simulink model "APV_ensemble_training"  (R2022a)
settings: Solver=VariableStepAuto  StartTime=0.0  StopTime=Tf  RelTol=1e-3  AbsTol=1e-4
InitFcn:
  | % show(map);
  | if doTraining == 0
  | setOccupied(map, 1:46);
  | setFree(map, freeSpotIndex);
  | end
values from neighbouring files (symbols this model uses):
  centerToRear = 1.343    [ParkingLotEnvironment.m]    (also in autoParkingValetParams3D.m)
  lidarTol = 0.2    [autoParkingValetParams3D.m]
  map = evalin('base',obj.MapObject)    [Camera.m]    (also in LIDARSensor.m = evalin('base', this.MapObject); ParkingLot2DVisualizer.m)
  maxLidarDist = 6    [autoParkingValetParams3D.m]
  numSensors = numel(lidar)    [ParkingLotEnvironment.m]    (also in autoParkingValetParams3D.m = 12)
  pTracking = 10    [createMPCForParking3D.m]
  speedMax = 2    [autoParkingValetParams3D.m]
  steerMax = pi/4    (= 0.785398163397)    [autoParkingValetParams3D.m]
  terrTol = deg2rad(10)    [autoParkingValetParams3D.m]
  trainXBounds = map.TrainingZoneXLimits    [autoParkingValetParams3D.m]
  trainYBounds = map.TrainingZoneYLimits    [autoParkingValetParams3D.m]
  Ts = 0.1    [createMPCForParking3D.m]
  xBounds = map.XLimits    [autoParkingValetParams3D.m]
  Xref = createReferenceTrajectory(Ts,Tf,freeSpotIndex)    [createMPCForParking3D.m]    (also in createReferenceTrajectory.m = [xRef(1:p,:);repmat(xRef(end,:),Tsteps-p,1)])
  xyerrTol = 0.75    [autoParkingValetParams3D.m]
  yBounds = map.YLimits    [autoParkingValetParams3D.m]
undefined symbols (not defined in the file or in its folder): actionTable, actionUB, collisionGain, distWeight, doTraining, egoInitialPose, egoTargetPose, freeSpotIndex, isTerminate, lidarGain, orientWeight, parkGain, rewardToIndex, rewardUB1, rewardUB2, stableWeight, stateTable, Tf, tranTable
libraries: rllib x10, mpclib x2, simulink x1, robotmobilelib x1, simulink_extras x1, sim3dlib x1, sim3dautolib x1
settings Model: PacingRate=0.089000  Creator=The MathWorks, Inc.  LastModifiedBy=momentumlab
settings SolverCC: AutoScaleAbsTol=off  AlgebraicLoopSolver=TrustRegion  MinimalZcImpactIntegration=on  MaxZcPerStep=1
settings DataIOCC: ReturnWorkspaceOutputs=off
settings DebuggingCC: UnconnectedInputMsg=warning  UnconnectedOutputMsg=warning  UnconnectedLineMsg=warning  SFMachineParentedDataDiag=warning
settings RTWCC: DLArmComputeVersion=19.05

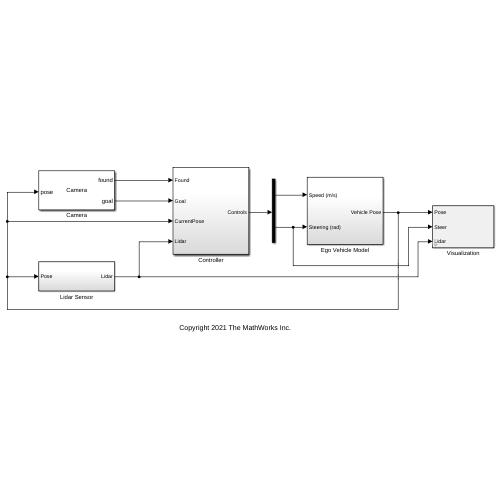
[thumbnail: Simulink's stored preview of the top-level diagram]
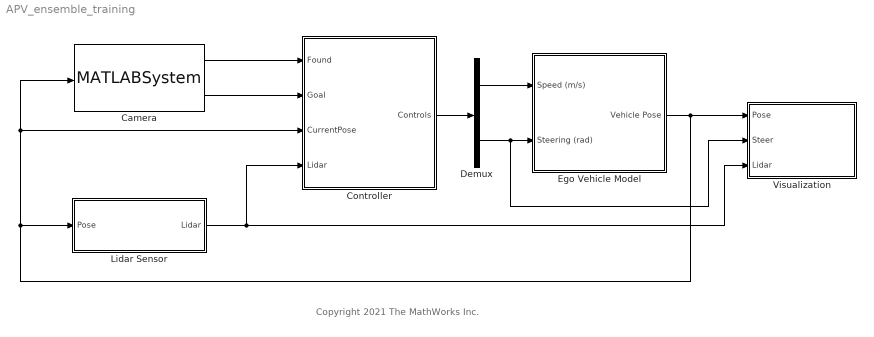
== system APV_ensemble_training ==
  note: Copyright 2021 The MathWorks Inc.
  Camera : MATLABSystem  System=Camera  MaxDepth=cameraDepth  MaxViewAngle=cameraViewAngle  MapObject=map
      mask Type: Camera
      mask Display:
      | disp('Camera');
      | port_label('input',1,'pose');
      | port_label('output',1,'found');
      | port_label('output',2,'goal');
  Controller : Subsystem
  Demux : Demux  Outputs=2
  Ego Vehicle Model : Subsystem
  Lidar Sensor : Subsystem
  Visualization : Subsystem  mask{doViz=Off, doVizUnreal=Off}
      mask prompts: doViz "2D Visualization"; doVizUnreal "Unreal Engine Visualization"
      mask TypeOptions doViz: Parking Lot 2D Visualization/doViz
      mask TypeOptions doVizUnreal: Unreal Engine Visualization/doVizUnreal
      mask DialogControl DescTextVar Prompt: Specify visualization options.
  wires:
  Demux/1 -> Ego Vehicle Model/1(Speed (m/s))
  Demux/2 -> Visualization/2(Steer), Ego Vehicle Model/2(Steering (rad))
  Lidar Sensor/1(Lidar) -> Visualization/3(Lidar), Controller/4(Lidar)
  Camera/1 -> Controller/1(Found)
  Camera/2 -> Controller/2(Goal)
  Controller/1(Controls) -> Demux/1
  Ego Vehicle Model/1(Vehicle Pose) -> Camera/1, Controller/3(CurrentPose), Lidar Sensor/1(Pose), Visualization/1(Pose)

== system APV_ensemble_training/Controller ==
  Found : Inport
  Goal : Inport  Port=2
  CurrentPose : Inport  Port=3
  Lidar : Inport  Port=4
  MPC Tracking Controller : Subsystem
  Merge : Merge
  RL Controller : Subsystem
  Vehicle Mode : Subsystem
  Controls : Outport
  wires:
  Merge/1 -> Controls/1
  CurrentPose/1 -> RL Controller/2(CurrentPose), MPC Tracking Controller/1(States)
  Vehicle Mode/3(TargetPose) -> RL Controller/1(Target)
  Lidar/1 -> RL Controller/3(Lidar)
  RL Controller/1(Actions) -> Merge/2
  MPC Tracking Controller/1(Controls) -> Merge/1
  Goal/1 -> Vehicle Mode/2(Goal)
  Found/1 -> Vehicle Mode/1(Found)
  Vehicle Mode/1(Search) -> MPC Tracking Controller/Enable
  Vehicle Mode/2(Park) -> RL Controller/Enable

== system APV_ensemble_training/Ego Vehicle Model ==
  Speed (m/s) : Inport
  Steering (rad) : Inport  Port=2
  Bicycle Kinematic Model : robotmobilelib/Bicycle Kinematic Model  VehicleInputs=Vehicle Speed & Steering Angle  WheelBase=map.centerToRear+map.centerToFront  VehicleSpeedRange=[-5, 5]  MaxSteeringAngle=steerMax  InitialState=egoInitialPose  SimulateUsing=Interpreted execution
      settings: SourceProductBaseCode=RO
  Demux : Demux  Outputs=3
  Ego Vehicle Pose : Scope  NumInputPorts=3
  Terminator : Terminator
  Vehicle Pose : Outport
  wires:
  Demux/3 -> Ego Vehicle Pose/3  "theta (rad)"
  Bicycle Kinematic Model/1 -> Demux/1, Vehicle Pose/1
  Demux/1 -> Ego Vehicle Pose/1  "x (m)"
  Bicycle Kinematic Model/2 -> Terminator/1
  Demux/2 -> Ego Vehicle Pose/2  "y (m)"
  Speed (m/s)/1 -> Bicycle Kinematic Model/1
  Steering (rad)/1 -> Bicycle Kinematic Model/2

== system APV_ensemble_training/Lidar Sensor ==
  Pose : Inport
  Demux : Demux  Outputs=3
  MATLAB System : MATLABSystem  System=LIDARSensor  MapObject=map  CarGeometry=map.VehicleDimensions  MaxDistance=maxLidarDist  SensorResolution=numSensors  ShowLIDARPlot=0  PlotLimits=[ xBounds yBounds ]
      mask Type: LIDARSensor
      mask Display:
      | disp('LIDARSensor');
      | port_label('input',1,'botx');
      | port_label('input',2,'boty');
      | port_label('input',3,'theta');
      | port_label('output',1,'d');
  Subsystem : Subsystem
  Lidar : Outport
  wires:
  Pose/1 -> Demux/1
  MATLAB System/1 -> Lidar/1
  Subsystem/1(centerX) -> MATLAB System/1
  Demux/2 -> Subsystem/2(currY)
  Demux/3 -> MATLAB System/3, Subsystem/3(theta)
  Demux/1 -> Subsystem/1(currX)
  Subsystem/2(centerY) -> MATLAB System/2

== system APV_ensemble_training/Visualization ==
  Pose : Inport
  Steer : Inport  Port=2
  Lidar : Inport  Port=3
  Parking Lot 2D Visualization : Subsystem  Variant=on  VariantControlMode=label  VariantControl=Choice  LabelModeActiveChoice=VizOff  mask{doViz=Off}
      mask prompts: doViz "2D Visualization"
      mask init:
      | choice = get_param(gcb,'doViz');
      | vssBlk = gcb;
      | if strcmp(choice,'On')
      |     set_param(vssBlk, 'LabelModeActiveChoice', 'VizOn');
      | else
      |     set_param(vssBlk, 'LabelModeActiveChoice', 'VizOff');
      | end
      mask TypeOptions doViz: On | Off
      mask DialogControl DescTextVar Tooltip: {"textId":"","text":""}
  Unreal Engine Visualization : Subsystem  Variant=on  VariantControlMode=label  VariantControl=Choice  LabelModeActiveChoice=UnrealOff  mask{doVizUnreal=Off}
      mask prompts: doVizUnreal "Unreal Engine Visualization"
      mask init:
      | choice = get_param(gcb,'doVizUnreal');
      | vssBlk = gcb;
      | if strcmp(choice,'On')
      |     set_param(vssBlk, 'LabelModeActiveChoice', 'UnrealOn');
      | else
      |     set_param(vssBlk, 'LabelModeActiveChoice', 'UnrealOff');
      | end
      mask TypeOptions doVizUnreal: On | Off
      mask DialogControl DescTextVar Tooltip: {"textId":"","text":""}
  wires:
  Pose/1 -> Unreal Engine Visualization/1(Pose), Parking Lot 2D Visualization/1(Pose)
  Steer/1 -> Parking Lot 2D Visualization/2(Steer)
  Lidar/1 -> Parking Lot 2D Visualization/3(Lidar)

== system APV_ensemble_training/Controller/MPC Tracking Controller ==
  States : Inport
  Enable : EnablePort  StatesWhenEnabling=reset
  Variant Subsystem : Subsystem  Variant=on  VariantControlMode=label  LabelModeActiveChoice=Choice_1  mask{choice=Adaptive MPC}
      mask init:
      | choice = get_param(gcb,'choice');
      | vssBlk = gcb;
      | oldVariant = get_param(gcb,'LabelModeActiveChoice');
      | if strcmp(choice,'Adaptive MPC')
      |     
      |     set_param(vssBlk, 'LabelModeActiveChoice', 'Choice_1');
      | else
      |     
      |     set_param(vssBlk, 'LabelModeActiveChoice', 'Choice_2');
      | end
      mask TypeOptions choice: Adaptive MPC | Nonlinear MPC
  Controls : Outport
  wires:
  States/1 -> Variant Subsystem/1(states)
  Variant Subsystem/1(controls) -> Controls/1

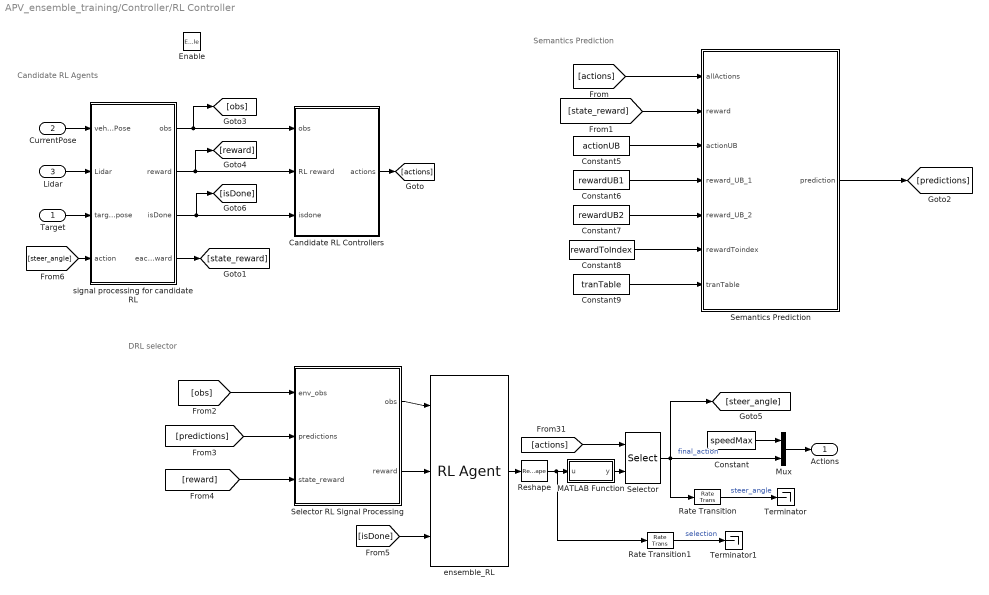
== system APV_ensemble_training/Controller/RL Controller ==
  note: Semantics Prediction
  note: Candidate RL Agents
  note: DRL selector
  Target : Inport
  CurrentPose : Inport  Port=2
  Lidar : Inport  Port=3
  Enable : EnablePort  StatesWhenEnabling=reset
  Candidate RL Controllers : Subsystem
  Constant : Constant  Value=speedMax
  Constant5 : Constant  Value=actionUB
  Constant6 : Constant  Value=rewardUB1
  Constant7 : Constant  Value=rewardUB2
  Constant8 : Constant  Value=rewardToIndex
  Constant9 : Constant  Value=tranTable
  MATLAB Function : MATLAB Function  TreatAsAtomicUnit=on
  Mux : Mux  Inputs=2
  Rate Transition : RateTransition  OutPortSampleTime=Ts_sample
  Rate Transition1 : RateTransition  OutPortSampleTime=Ts_sample
  Reshape : Reshape
  Selector : Selector  IndexOptions=Index vector (port)  Indices=[1 3]  OutputSizes=1
  Selector RL Signal Processing : Subsystem
  Semantics Prediction : Subsystem
  Terminator : Terminator
  Terminator1 : Terminator
  ensemble_RL : rllib/RL Agent  Agent=agentEnsemble  ExternalActionAsInput=off  ProvideLastAction=off  ProvideCumRwd=off  TreatAsDirectFeedthrough=on  UseStrictObservationDataTypes=off
  signal processing for candidate RL : Subsystem
  Actions : Outport
  wires:
  signal processing for candidate RL/1(obs) -> Candidate RL Controllers/1(obs), [obs]
  signal processing for candidate RL/2(reward) -> Candidate RL Controllers/2(RL reward), [reward]
  CurrentPose/1 -> signal processing for candidate RL/1(vehiclePose)
  Target/1 -> signal processing for candidate RL/3(targetpose)
  Lidar/1 -> signal processing for candidate RL/2(Lidar)
  Constant/1 -> Mux/1
  Mux/1 -> Actions/1
  signal processing for candidate RL/3(isDone) -> [isDone], Candidate RL Controllers/3(isdone)
  Rate Transition/1 -> Terminator/1  "steer_angle"
  Constant6/1 -> Semantics Prediction/4(reward_UB_1)
  Constant7/1 -> Semantics Prediction/5(reward_UB_2)
  Constant5/1 -> Semantics Prediction/3(actionUB)
  Constant9/1 -> Semantics Prediction/7(tranTable)
  [actions] -> Semantics Prediction/1(allActions)
  Constant8/1 -> Semantics Prediction/6(rewardToindex)
  Semantics Prediction/1(prediction) -> [predictions]
  [state_reward] -> Semantics Prediction/2(reward)
  Candidate RL Controllers/1(actions) -> [actions]
  [isDone] -> ensemble_RL/3
  Reshape/1 -> Rate Transition1/1, MATLAB Function/1(u)
  Selector/1 -> Rate Transition/1, Mux/2, [steer_angle]  "final_action"
  [predictions] -> Selector RL Signal Processing/2(predictions)
  Selector RL Signal Processing/2(reward) -> ensemble_RL/2
  [actions] -> Selector/1
  Selector RL Signal Processing/1(obs) -> ensemble_RL/1
  [obs] -> Selector RL Signal Processing/1(env_obs)
  [reward] -> Selector RL Signal Processing/3(state_reward)
  signal processing for candidate RL/4(each_reward) -> [state_reward]
  [steer_angle] -> signal processing for candidate RL/4(action)
  Rate Transition1/1 -> Terminator1/1  "selection"
  ensemble_RL/1 -> Reshape/1
  MATLAB Function/1(y) -> Selector/2

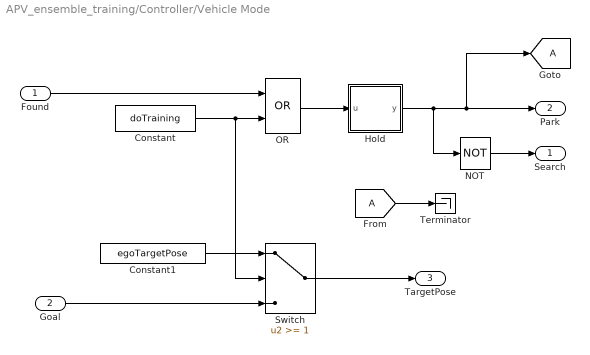
== system APV_ensemble_training/Controller/Vehicle Mode ==
  Found : Inport
  Goal : Inport  Port=2
  Constant : Constant  Value=doTraining
  Constant1 : Constant  Value=egoTargetPose
  From : From  TagVisibility=global
  Goto : Goto  TagVisibility=global
  Hold : Subsystem
  NOT : Logic  Operator=NOT  AllPortsSameDT=off  OutDataTypeStr=boolean
  OR : Logic  Operator=OR  AllPortsSameDT=off  OutDataTypeStr=boolean
  Switch : Switch  Threshold=1  SaturateOnIntegerOverflow=off  InputSameDT=off
  Terminator : Terminator
  Search : Outport
  Park : Outport  Port=2
  TargetPose : Outport  Port=3
  wires:
  Found/1 -> OR/1
  OR/1 -> Hold/1(u)
  NOT/1 -> Search/1
  Hold/1(y) -> Goto/1, Park/1, NOT/1
  Constant1/1 -> Switch/1
  Switch/1 -> TargetPose/1
  Constant/1 -> Switch/2, OR/2
  Goal/1 -> Switch/3
  From/1 -> Terminator/1

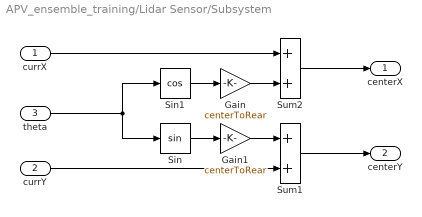
== system APV_ensemble_training/Lidar Sensor/Subsystem ==
  currX : Inport
  currY : Inport  Port=2
  theta : Inport  Port=3
  Gain : Gain  Gain=centerToRear
  Gain1 : Gain  Gain=centerToRear
  Sin : Trigonometry
  Sin1 : Trigonometry  Operator=cos
  Sum1 : Sum
  Sum2 : Sum
  centerX : Outport
  centerY : Outport  Port=2
  wires:
  Sum1/1 -> centerY/1
  currY/1 -> Sum1/2
  theta/1 -> Sin/1, Sin1/1
  Sin/1 -> Gain1/1
  Sin1/1 -> Gain/1
  currX/1 -> Sum2/1
  Sum2/1 -> centerX/1
  Gain/1 -> Sum2/2
  Gain1/1 -> Sum1/1

== system APV_ensemble_training/Visualization/Parking Lot 2D Visualization ==
  Pose : Inport
  Steer : Inport  Port=2
  Lidar : Inport  Port=3
  Off : Subsystem  VariantControl=VizOff
  On : Subsystem  VariantControl=VizOn

== system APV_ensemble_training/Visualization/Unreal Engine Visualization ==
  Pose : Inport
  Off : Subsystem  VariantControl=UnrealOff
  On : Subsystem  VariantControl=UnrealOn

== system APV_ensemble_training/Controller/MPC Tracking Controller/Variant Subsystem ==
  note: 1) Add Subsystem or Model blocks as valid variant choices.
      | 2) You cannot connect blocks at this level. At simulation, connectivity is automatically
      | determined, based on the active variant and port name matching.
  states : Inport
  Adaptive MPC : Subsystem  VariantControl=Choice_1
  Nonlinear MPC : Subsystem  VariantControl=Choice_2
  controls : Outport

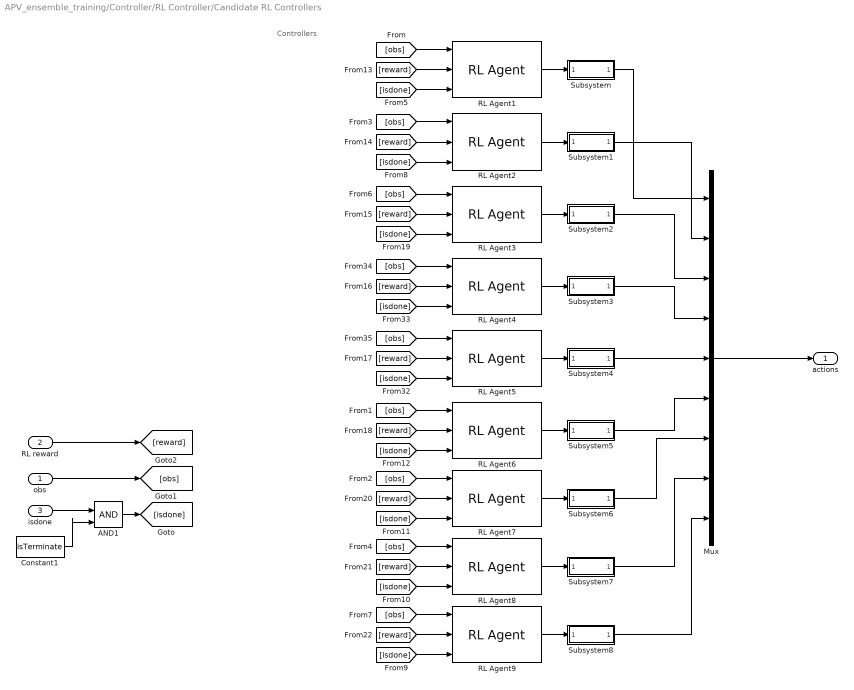
== system APV_ensemble_training/Controller/RL Controller/Candidate RL Controllers ==
  note: Controllers
  obs : Inport
  RL reward : Inport  Port=2
  isdone : Inport  Port=3
  AND1 : Logic  IconShape=distinctive  AllPortsSameDT=off  OutDataTypeStr=boolean
  Constant1 : Constant  Value=isTerminate
  Mux : Mux  Inputs=9
  RL Agent1 : rllib/RL Agent  Agent=agent1  ExternalActionAsInput=off  ProvideLastAction=off  ProvideCumRwd=off  TreatAsDirectFeedthrough=on  UseStrictObservationDataTypes=off
  RL Agent2 : rllib/RL Agent  Agent=agent2  ExternalActionAsInput=off  ProvideLastAction=off  ProvideCumRwd=off  TreatAsDirectFeedthrough=on  UseStrictObservationDataTypes=off
  RL Agent3 : rllib/RL Agent  Agent=agent3  ExternalActionAsInput=off  ProvideLastAction=off  ProvideCumRwd=off  TreatAsDirectFeedthrough=on  UseStrictObservationDataTypes=off
  RL Agent4 : rllib/RL Agent  Agent=agent3  ExternalActionAsInput=off  ProvideLastAction=off  ProvideCumRwd=off  TreatAsDirectFeedthrough=on  UseStrictObservationDataTypes=off
  RL Agent5 : rllib/RL Agent  Agent=agent3  ExternalActionAsInput=off  ProvideLastAction=off  ProvideCumRwd=off  TreatAsDirectFeedthrough=on  UseStrictObservationDataTypes=off
  RL Agent6 : rllib/RL Agent  Agent=agent6  ExternalActionAsInput=off  ProvideLastAction=off  ProvideCumRwd=off  TreatAsDirectFeedthrough=on  UseStrictObservationDataTypes=off
  RL Agent7 : rllib/RL Agent  Agent=agent7  ExternalActionAsInput=off  ProvideLastAction=off  ProvideCumRwd=off  TreatAsDirectFeedthrough=on  UseStrictObservationDataTypes=off
  RL Agent8 : rllib/RL Agent  Agent=agent8  ExternalActionAsInput=off  ProvideLastAction=off  ProvideCumRwd=off  TreatAsDirectFeedthrough=on  UseStrictObservationDataTypes=off
  RL Agent9 : rllib/RL Agent  Agent=agent9  ExternalActionAsInput=off  ProvideLastAction=off  ProvideCumRwd=off  TreatAsDirectFeedthrough=on  UseStrictObservationDataTypes=off
  Subsystem : Subsystem
  Subsystem1 : Subsystem
  Subsystem2 : Subsystem
  Subsystem3 : Subsystem
  Subsystem4 : Subsystem
  Subsystem5 : Subsystem
  Subsystem6 : Subsystem
  Subsystem7 : Subsystem
  Subsystem8 : Subsystem
  actions : Outport
  wires:
  [obs] -> RL Agent7/1
  [obs] -> RL Agent4/1
  [obs] -> RL Agent3/1
  Subsystem3/1(action) -> Mux/4
  [obs] -> RL Agent1/1
  [isdone] -> RL Agent1/3
  [obs] -> RL Agent2/1
  [obs] -> RL Agent5/1
  RL Agent1/1 -> Subsystem/1(rlOut)
  [isdone] -> RL Agent8/3
  [isdone] -> RL Agent6/3
  Subsystem/1(action) -> Mux/1
  RL Agent6/1 -> Subsystem5/1(rlOut)
  Subsystem4/1(action) -> Mux/5
  RL Agent3/1 -> Subsystem2/1(rlOut)
  [isdone] -> RL Agent2/3
  [isdone] -> RL Agent7/3
  RL Agent8/1 -> Subsystem7/1(rlOut)
  Subsystem1/1(action) -> Mux/2
  [isdone] -> RL Agent5/3
  Mux/1 -> actions/1
  [obs] -> RL Agent6/1
  [isdone] -> RL Agent3/3
  RL Agent5/1 -> Subsystem4/1(rlOut)
  RL Agent4/1 -> Subsystem3/1(rlOut)
  RL Agent7/1 -> Subsystem6/1(rlOut)
  RL Agent2/1 -> Subsystem1/1(rlOut)
  [obs] -> RL Agent8/1
  Subsystem2/1(action) -> Mux/3
  [isdone] -> RL Agent4/3
  RL Agent9/1 -> Subsystem8/1(rlOut)
  [obs] -> RL Agent9/1
  [isdone] -> RL Agent9/3
  Subsystem5/1(action) -> Mux/6
  Subsystem6/1(action) -> Mux/7
  Subsystem7/1(action) -> Mux/8
  Subsystem8/1(action) -> Mux/9
  obs/1 -> [obs]
  RL reward/1 -> [reward]
  [reward] -> RL Agent1/2
  [reward] -> RL Agent2/2
  [reward] -> RL Agent3/2
  [reward] -> RL Agent4/2
  [reward] -> RL Agent5/2
  [reward] -> RL Agent6/2
  [reward] -> RL Agent7/2
  [reward] -> RL Agent8/2
  [reward] -> RL Agent9/2
  AND1/1 -> [isdone]
  isdone/1 -> AND1/1
  Constant1/1 -> AND1/2

== system APV_ensemble_training/Controller/RL Controller/Selector RL Signal Processing ==
  env_obs : Inport
  predictions : Inport  Port=2
  state_reward : Inport  Port=3
  Mux : Mux  Inputs=2
  Terminator : Terminator
  obs : Outport
  reward : Outport  Port=2
  wires:
  state_reward/1 -> reward/1
  predictions/1 -> Mux/2
  env_obs/1 -> Mux/1
  Mux/1 -> obs/1, Terminator/1

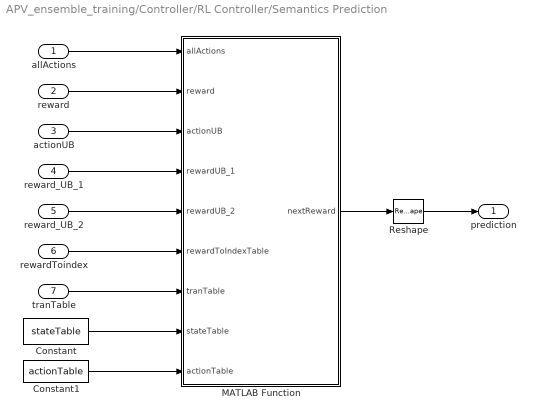
== system APV_ensemble_training/Controller/RL Controller/Semantics Prediction ==
  allActions : Inport
  reward : Inport  Port=2
  actionUB : Inport  Port=3
  reward_UB_1 : Inport  Port=4
  reward_UB_2 : Inport  Port=5
  rewardToindex : Inport  Port=6
  tranTable : Inport  Port=7
  Constant : Constant  Value=stateTable
  Constant1 : Constant  Value=actionTable
  MATLAB Function : MATLAB Function  TreatAsAtomicUnit=on
  Reshape : Reshape
  prediction : Outport
  wires:
  MATLAB Function/1(nextReward) -> Reshape/1
  allActions/1 -> MATLAB Function/1(allActions)
  reward/1 -> MATLAB Function/2(reward)
  actionUB/1 -> MATLAB Function/3(actionUB)
  reward_UB_1/1 -> MATLAB Function/4(rewardUB_1)
  reward_UB_2/1 -> MATLAB Function/5(rewardUB_2)
  rewardToindex/1 -> MATLAB Function/6(rewardToIndexTable)
  tranTable/1 -> MATLAB Function/7(tranTable)
  Constant/1 -> MATLAB Function/8(stateTable)
  Constant1/1 -> MATLAB Function/9(actionTable)
  Reshape/1 -> prediction/1

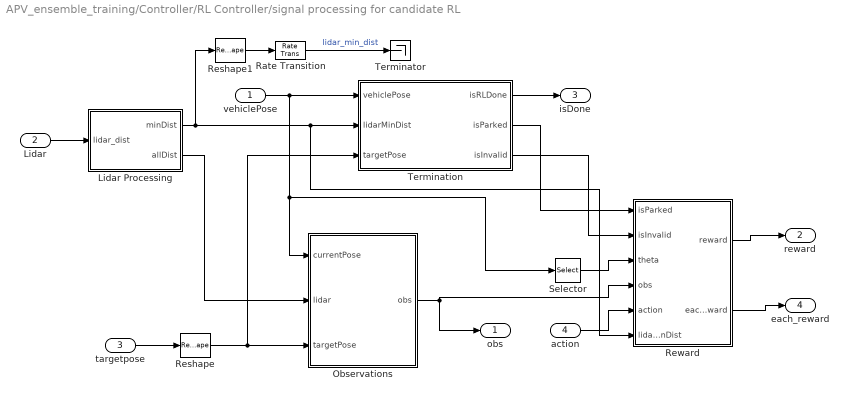
== system APV_ensemble_training/Controller/RL Controller/signal processing for candidate RL ==
  vehiclePose : Inport
  Lidar : Inport  Port=2
  targetpose : Inport  Port=3
  action : Inport  Port=4
  Lidar Processing : Subsystem
  Observations : Subsystem
  Rate Transition : RateTransition  OutPortSampleTime=Ts_sample
  Reshape : Reshape
  Reshape1 : Reshape
  Reward : Subsystem
  Selector : Selector  InputPortWidth=3  IndexOptions=Index vector (dialog)  Indices=3  OutputSizes=1
  Termination : Subsystem
  Terminator : Terminator
  obs : Outport
  reward : Outport  Port=2
  isDone : Outport  Port=3
  each_reward : Outport  Port=4
  wires:
  action/1 -> Reward/5(action)
  Reward/1(reward) -> reward/1
  targetpose/1 -> Reshape/1
  Lidar Processing/1(minDist) -> Reshape1/1, Reward/6(lidarMinDist), Termination/2(lidarMinDist)
  Lidar Processing/2(allDist) -> Observations/2(lidar)
  vehiclePose/1 -> Observations/1(currentPose), Selector/1, Termination/1(vehiclePose)
  Observations/1(obs) -> obs/1, Reward/4(obs)
  Lidar/1 -> Lidar Processing/1(lidar_dist)
  Selector/1 -> Reward/3(theta)
  Termination/2(isParked) -> Reward/1(isParked)
  Reshape/1 -> Termination/3(targetPose), Observations/3(targetPose)
  Termination/1(isRLDone) -> isDone/1
  Termination/3(isInvalid) -> Reward/2(isInvalid)
  Rate Transition/1 -> Terminator/1  "lidar_min_dist"
  Reshape1/1 -> Rate Transition/1
  Reward/2(each_reward) -> each_reward/1

== system APV_ensemble_training/Controller/Vehicle Mode/Hold ==
  u : Inport
  Add : Sum
  Data Type Conversion : DataTypeConversion  OutDataTypeStr=boolean  SaturateOnIntegerOverflow=off  RndMeth=Floor
  Data Type Conversion2 : DataTypeConversion  OutDataTypeStr=double  SaturateOnIntegerOverflow=off  RndMeth=Floor
  Memory : Memory
  Saturation : Saturate  UpperLimit=1  LowerLimit=0
  y : Outport
  wires:
  u/1 -> Data Type Conversion2/1
  Add/1 -> Saturation/1, Memory/1
  Memory/1 -> Add/2
  Saturation/1 -> Data Type Conversion/1
  Data Type Conversion/1 -> y/1
  Data Type Conversion2/1 -> Add/1

== system APV_ensemble_training/Visualization/Parking Lot 2D Visualization/Off ==
  Pose : Inport
  Steer : Inport  Port=2
  Lidar : Inport  Port=3
  Terminator : Terminator
  Terminator1 : Terminator
  Terminator2 : Terminator
  wires:
  Lidar/1 -> Terminator2/1
  Pose/1 -> Terminator/1
  Steer/1 -> Terminator1/1

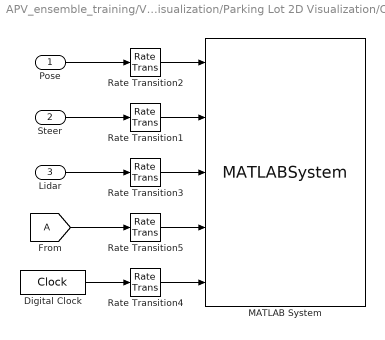
== system APV_ensemble_training/Visualization/Parking Lot 2D Visualization/On ==
  Pose : Inport
  Steer : Inport  Port=2
  Lidar : Inport  Port=3
  Digital Clock : DigitalClock  SampleTime=Ts
  From : From  TagVisibility=global
  MATLAB System : MATLABSystem  System=ParkingLot2DVisualizer  MapObject=map  CameraDepth=10  CameraViewAngle=deg2rad(60)  MaxLidarDistance=6  TrainingFlag=doTraining
      mask Type: ParkingLot2DVisualizer
      mask Display:
      | disp('ParkingLot2DVisualizer');
      | port_label('input',1,'pose');
      | port_label('input',2,'steer');
      | port_label('input',3,'lidar');
      | port_label('input',4,'park');
      | port_label('input',5,'currentTime');
  Rate Transition{1..5} (5 alike) : RateTransition
  wires:
  Steer/1 -> Rate Transition1/1
  Pose/1 -> Rate Transition2/1
  Rate Transition1/1 -> MATLAB System/2
  Lidar/1 -> Rate Transition3/1
  From/1 -> Rate Transition5/1
  Digital Clock/1 -> Rate Transition4/1
  Rate Transition4/1 -> MATLAB System/5
  Rate Transition2/1 -> MATLAB System/1
  Rate Transition3/1 -> MATLAB System/3
  Rate Transition5/1 -> MATLAB System/4

== system APV_ensemble_training/Visualization/Unreal Engine Visualization/Off ==
  Pose : Inport
  Terminator : Terminator
  wires:
  Pose/1 -> Terminator/1

== system APV_ensemble_training/Visualization/Unreal Engine Visualization/On ==
  Pose : Inport
  Demux1 : Demux  Outputs=3
  Radians to Degrees : simulink_extras/Transformations/Radians to Degrees
  Simulation 3D Scene Configuration : sim3dlib/Simulation 3D Scene Configuration  Priority=0  ProjectFormat=Default Scenes  SceneDesc=Large parking lot  ProjectName=/home/momentumlab/Documents/MATLAB/R2022a/toolbox/shared/sim3d_projects/automotive_project/UE4/LinuxNoEditor/AutoVrtlEnv.sh  ScenePath=/Game/Maps/HwStrght  vehTagList={'Scene Origin';'SimulinkVehicle1'}  vehTag=SimulinkVehicle1  OpVisEn=off  Ts=Ts  EnableWindow=on  EnableRemoteAccess=off  EnableWeather=off  SunAltitude=40.0  SunAzimuth=90  clouds=10  wind=1  fog=0  rain=0  sensorTag=MainCamera1  sensorId=1  sensorName=MainCamera1  mountLoc=Origin  offsetFlag=off  tmountOffset=[0, 0, 0]  rmountOffset=[0, 0, 0]  HorizontalResolution=1280  VerticalResolution=720  HorizontalFOV=60  mountPoint=[0 0 0]  mountOrientation=[0 0 0]  aMode=3  ID=1
      settings: SourceProductBaseCode=VE,AE,DR,UV,VE
  Simulation 3D Vehicle with Ground Following : sim3dautolib/Simulation 3D Vehicle with Ground Following  Priority=-1  PassVehMesh=Hatchback  MeshPath=/MathWorksSimulation/Vehicles/Muscle/Meshes/SK_MuscleCar.SK_MuscleCar  TrackWidth=1.9  WheelBase=3  WheelRadius=0.35  VehColor=Red  InitialPos=[egoInitialPose(1)+cos(egoInitialPose(3))*centerToRear, egoInitialPose(2)+sin(egoInitialPose(3))*centerToRear, 0]  InitialRot=[0, 0, rad2deg(egoInitialPose(3))]  ActorName=SimulinkVehicle1  SampleTime=-1  ActorType=SimulinkVehicle  ID=1  aMode=3  ActorTag=SimulinkVehicle1  CoordinateScheme=ISO  VehLightsControl=off  HeadlightColor=[ 1, 1, 1 ]  HighBeamIntensity=100000  LowBeamIntensity=60000  HighBeamConeAngle=70  LowBeamConeAngle=70  LeftHeadlightOrientation=[ 0, 0 ]  RightHeadlightOrientation=[ 0, 0 ]  BrakelightIntensity=500  ReverselightIntensity=500  SignallightIntensity=500  SignallightPeriod=1  SignalPulseWidth=50  TransformOutportEnabled=off
      settings: SourceProductBaseCode=VE,AE,DR,UV,VE
  wires:
  Pose/1 -> Demux1/1
  Demux1/3 -> Radians to Degrees/1
  Demux1/2 -> Simulation 3D Vehicle with Ground Following/2
  Demux1/1 -> Simulation 3D Vehicle with Ground Following/1
  Radians to Degrees/1 -> Simulation 3D Vehicle with Ground Following/3

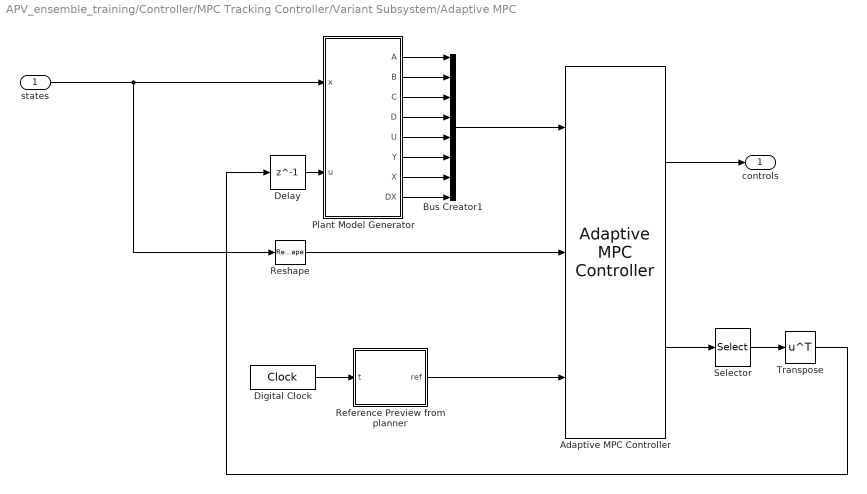
== system APV_ensemble_training/Controller/MPC Tracking Controller/Variant Subsystem/Adaptive MPC ==
  states : Inport
  Adaptive MPC Controller : mpclib/Adaptive MPC Controller  SCDEnableBlockLinearizationSpecification=on  mpcobj=mpcobj  enable_value=0  updateMPCinCallerWorkspace=on  md_inport=off  mv_inport=off  uref_inport=off  return_cost=off  return_mvseq=on  return_qpstatus=off  return_xseq=off  return_state=off  return_ovseq=off  state_inport=on  isltv_plant=off  umin_inport=off  umax_inport=off  ymin_inport=off  ymax_inport=off  cc_inport=off  ywt_inport=off  uwt_inport=off  duwt_inport=off  rhoeps_inport=off  pm_inport=off  MaximumP=10  HorizonChoice=FixedHorizon  BlockDataType=double  SampleTimeInherited=off  switch_inport=off
  Bus Creator1 : BusCreator  Inputs=8
  Delay : Delay  DelayLength=1
  Digital Clock : DigitalClock  SampleTime=Ts
  Plant Model Generator : MATLAB Function  TreatAsAtomicUnit=on
  Reference Preview from planner : MATLAB Function  TreatAsAtomicUnit=on
  Reshape : Reshape  OutputDimensionality=Customize  OutputDimensions=[3,1]
  Selector : Selector  NumberOfDimensions=2  InputPortWidth=3  IndexOptions=Index vector (dialog),Select all  Indices=2,2  OutputSizes=1,1
  Transpose : Math  Operator=transpose  SignedPower=on
  controls : Outport
  wires:
  Adaptive MPC Controller/1 -> controls/1
  Selector/1 -> Transpose/1
  Delay/1 -> Plant Model Generator/2(u)
  Reshape/1 -> Adaptive MPC Controller/2
  Plant Model Generator/1(A) -> Bus Creator1/1
  Plant Model Generator/6(Y) -> Bus Creator1/6
  Transpose/1 -> Delay/1
  Plant Model Generator/3(C) -> Bus Creator1/3
  states/1 -> Reshape/1, Plant Model Generator/1(x)
  Plant Model Generator/8(DX) -> Bus Creator1/8
  Reference Preview from planner/1(ref) -> Adaptive MPC Controller/3
  Plant Model Generator/2(B) -> Bus Creator1/2
  Plant Model Generator/5(U) -> Bus Creator1/5
  Adaptive MPC Controller/2 -> Selector/1
  Plant Model Generator/4(D) -> Bus Creator1/4
  Plant Model Generator/7(X) -> Bus Creator1/7
  Digital Clock/1 -> Reference Preview from planner/1(t)
  Bus Creator1/1 -> Adaptive MPC Controller/1

== system APV_ensemble_training/Controller/MPC Tracking Controller/Variant Subsystem/Nonlinear MPC ==
  states : Inport
  Delay : Delay  DelayLength=1
  Digital Clock : DigitalClock  SampleTime=Ts
  Nonlinear MPC Controller : mpclib/Nonlinear MPC Controller  SCDEnableBlockLinearizationSpecification=on  nlmpcobj=nlobjTracking  UseObjectTs=on  UseMEX=off  md_enabled=off  mvtarget_enabled=off  param_enabled=off  cost_enabled=off  mvseq_enabled=off  stateseq_enabled=off  ovseq_enabled=off  slack_enabled=off  status_enabled=off  ov_min=off  ov_max=off  mv_min=off  mv_max=off  mvrate_min=off  mvrate_max=off  state_min=off  state_max=off  ov_weight=off  mv_weight=off  mvrate_weight=off  ecr_weight=off  nlp_initialize=off
  Reference Preview from RRT : MATLAB Function  TreatAsAtomicUnit=on
  Reshape : Reshape  OutputDimensionality=Customize  OutputDimensions=[2,1]
  controls : Outport
  wires:
  Reference Preview from RRT/1(ref) -> Nonlinear MPC Controller/2
  Digital Clock/1 -> Reference Preview from RRT/1(t)
  Delay/1 -> Nonlinear MPC Controller/3
  states/1 -> Nonlinear MPC Controller/1
  Reshape/1 -> controls/1, Delay/1
  Nonlinear MPC Controller/1 -> Reshape/1

== system APV_ensemble_training/Controller/RL Controller/Candidate RL Controllers/Subsystem ==
  rlOut : Inport
  Gain : Gain  Gain=steerMax
  Reshape : Reshape
  Saturation9 : Saturate  UpperLimit=steerMax  LowerLimit=-steerMax
  action : Outport
  wires:
  Saturation9/1 -> action/1
  rlOut/1 -> Gain/1
  Gain/1 -> Reshape/1
  Reshape/1 -> Saturation9/1

== system APV_ensemble_training/Controller/RL Controller/Candidate RL Controllers/Subsystem1 ==
  rlOut : Inport
  Gain : Gain  Gain=steerMax
  Reshape : Reshape
  Saturation9 : Saturate  UpperLimit=steerMax  LowerLimit=-steerMax
  action : Outport
  wires:
  Saturation9/1 -> action/1
  rlOut/1 -> Gain/1
  Gain/1 -> Reshape/1
  Reshape/1 -> Saturation9/1

== system APV_ensemble_training/Controller/RL Controller/Candidate RL Controllers/Subsystem2 ==
  rlOut : Inport
  Gain : Gain  Gain=steerMax
  Reshape : Reshape
  Saturation9 : Saturate  UpperLimit=steerMax  LowerLimit=-steerMax
  action : Outport
  wires:
  Saturation9/1 -> action/1
  rlOut/1 -> Gain/1
  Gain/1 -> Reshape/1
  Reshape/1 -> Saturation9/1

== system APV_ensemble_training/Controller/RL Controller/Candidate RL Controllers/Subsystem3 ==
  rlOut : Inport
  Gain : Gain  Gain=steerMax
  Reshape : Reshape
  Saturation9 : Saturate  UpperLimit=steerMax  LowerLimit=-steerMax
  action : Outport
  wires:
  Saturation9/1 -> action/1
  rlOut/1 -> Gain/1
  Gain/1 -> Reshape/1
  Reshape/1 -> Saturation9/1

== system APV_ensemble_training/Controller/RL Controller/Candidate RL Controllers/Subsystem4 ==
  rlOut : Inport
  Gain : Gain  Gain=steerMax
  Reshape : Reshape
  Saturation9 : Saturate  UpperLimit=steerMax  LowerLimit=-steerMax
  action : Outport
  wires:
  Saturation9/1 -> action/1
  rlOut/1 -> Gain/1
  Gain/1 -> Reshape/1
  Reshape/1 -> Saturation9/1

== system APV_ensemble_training/Controller/RL Controller/Candidate RL Controllers/Subsystem5 ==
  rlOut : Inport
  Gain : Gain  Gain=steerMax
  Reshape : Reshape
  Saturation9 : Saturate  UpperLimit=steerMax  LowerLimit=-steerMax
  action : Outport
  wires:
  Saturation9/1 -> action/1
  rlOut/1 -> Gain/1
  Gain/1 -> Reshape/1
  Reshape/1 -> Saturation9/1

== system APV_ensemble_training/Controller/RL Controller/Candidate RL Controllers/Subsystem6 ==
  rlOut : Inport
  Gain : Gain  Gain=steerMax
  Reshape : Reshape
  Saturation9 : Saturate  UpperLimit=steerMax  LowerLimit=-steerMax
  action : Outport
  wires:
  Saturation9/1 -> action/1
  rlOut/1 -> Gain/1
  Gain/1 -> Reshape/1
  Reshape/1 -> Saturation9/1

== system APV_ensemble_training/Controller/RL Controller/Candidate RL Controllers/Subsystem7 ==
  rlOut : Inport
  Gain : Gain  Gain=steerMax
  Reshape : Reshape
  Saturation9 : Saturate  UpperLimit=steerMax  LowerLimit=-steerMax
  action : Outport
  wires:
  Saturation9/1 -> action/1
  rlOut/1 -> Gain/1
  Gain/1 -> Reshape/1
  Reshape/1 -> Saturation9/1

== system APV_ensemble_training/Controller/RL Controller/Candidate RL Controllers/Subsystem8 ==
  rlOut : Inport
  Gain : Gain  Gain=steerMax
  Reshape : Reshape
  Saturation9 : Saturate  UpperLimit=steerMax  LowerLimit=-steerMax
  action : Outport
  wires:
  Saturation9/1 -> action/1
  rlOut/1 -> Gain/1
  Gain/1 -> Reshape/1
  Reshape/1 -> Saturation9/1

== system APV_ensemble_training/Controller/RL Controller/signal processing for candidate RL/Lidar Processing ==
  lidar_dist : Inport
  MATLAB Function : MATLAB Function  TreatAsAtomicUnit=on  mask{Res=numSensors, LW=map.VehicleDimensions}
      mask prompts: Res "Number of available measurements"; LW "Geometry of the car [L,W]"
      mask init:
      | res = Res;
      | L = LW(1);W = LW(2);
  MinMax : MinMax
  Sum : Sum  Inputs=|+-
  minDist : Outport
  allDist : Outport  Port=2
  wires:
  Sum/1 -> MinMax/1
  MATLAB Function/1(carDistances) -> Sum/2
  MinMax/1 -> minDist/1
  lidar_dist/1 -> Sum/1, allDist/1

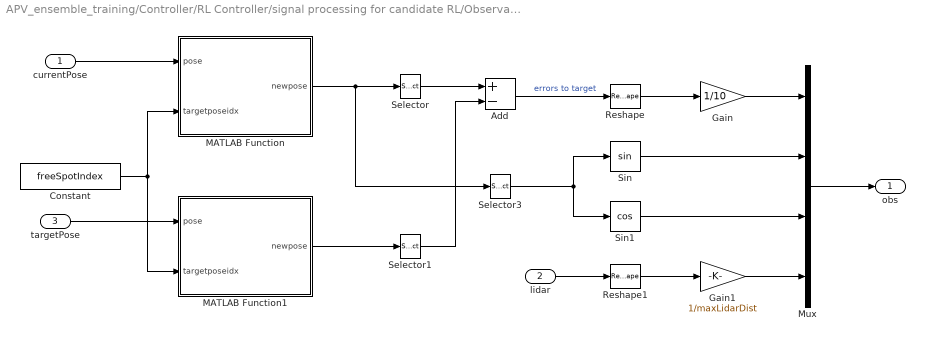
== system APV_ensemble_training/Controller/RL Controller/signal processing for candidate RL/Observations ==
  currentPose : Inport
  lidar : Inport  Port=2
  targetPose : Inport  Port=3
  Add : Sum  Inputs=+-
  Constant : Constant  Value=freeSpotIndex
  Gain : Gain  Gain=1/10
  Gain1 : Gain  Gain=1/maxLidarDist
  MATLAB Function : MATLAB Function  TreatAsAtomicUnit=on
  MATLAB Function1 : MATLAB Function  TreatAsAtomicUnit=on
  Mux : Mux
  Reshape : Reshape
  Reshape1 : Reshape
  Selector : Selector  InputPortWidth=3  IndexOptions=Index vector (dialog)  Indices=1:2  OutputSizes=1
  Selector1 : Selector  InputPortWidth=3  IndexOptions=Index vector (dialog)  Indices=1:2  OutputSizes=1
  Selector3 : Selector  InputPortWidth=3  IndexOptions=Index vector (dialog)  Indices=3  OutputSizes=1
  Sin : Trigonometry
  Sin1 : Trigonometry  Operator=cos
  obs : Outport
  wires:
  Reshape/1 -> Gain/1
  Add/1 -> Reshape/1  "errors to target"
  lidar/1 -> Reshape1/1
  Mux/1 -> obs/1
  Reshape1/1 -> Gain1/1
  Selector/1 -> Add/1
  Selector1/1 -> Add/2
  Sin/1 -> Mux/2
  Sin1/1 -> Mux/3
  Selector3/1 -> Sin/1, Sin1/1
  Gain/1 -> Mux/1
  Gain1/1 -> Mux/4
  currentPose/1 -> MATLAB Function/1(pose)
  targetPose/1 -> MATLAB Function1/1(pose)
  Constant/1 -> MATLAB Function/2(targetposeidx), MATLAB Function1/2(targetposeidx)
  MATLAB Function/1(newpose) -> Selector3/1, Selector/1
  MATLAB Function1/1(newpose) -> Selector1/1

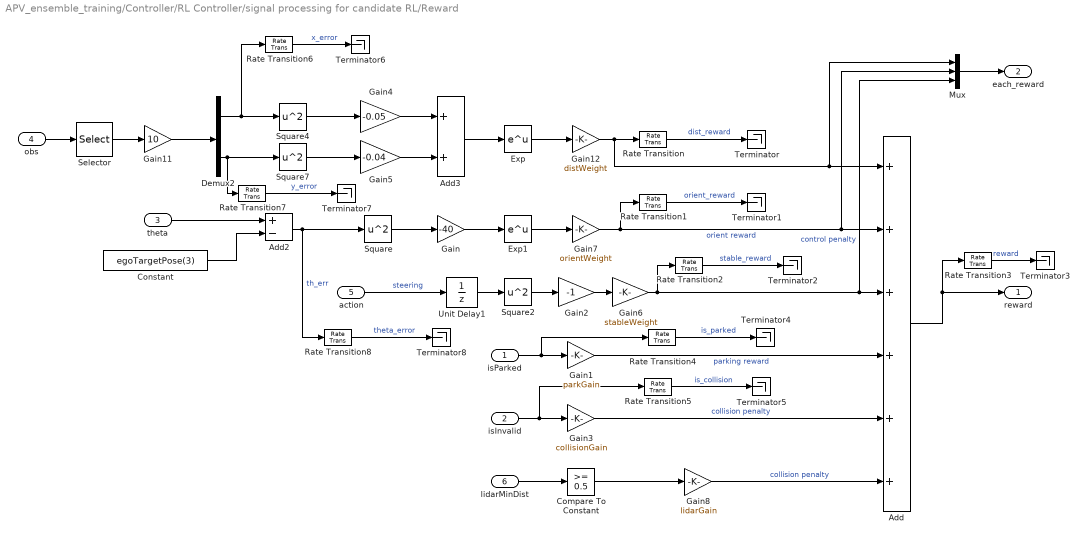
== system APV_ensemble_training/Controller/RL Controller/signal processing for candidate RL/Reward ==
  isParked : Inport
  isInvalid : Inport  Port=2
  theta : Inport  Port=3
  obs : Inport  Port=4
  action : Inport  Port=5
  lidarMinDist : Inport  Port=6
  Add : Sum  Inputs=++++++
  Add2 : Sum  Inputs=+-
  Add3 : Sum
  Compare To Constant : simulink/Logic and Bit Operations/Compare To Constant  relop=>=  const=0.5  OutDataTypeStr=boolean
  Constant : Constant  Value=egoTargetPose(3)
  Demux2 : Demux  Outputs=2
  Exp : Math
  Exp1 : Math
  Gain : Gain  Gain=-40
  Gain1 : Gain  Gain=parkGain
  Gain11 : Gain  Gain=10
  Gain12 : Gain  Gain=distWeight
  Gain2 : Gain  Gain=-1
  Gain3 : Gain  Gain=collisionGain
  Gain4 : Gain  Gain=-0.05
  Gain5 : Gain  Gain=-0.04
  Gain6 : Gain  Gain=stableWeight
  Gain7 : Gain  Gain=orientWeight
  Gain8 : Gain  Gain=lidarGain
  Mux : Mux  Inputs=3
  Rate Transition{,1..8} (9 alike) : RateTransition  OutPortSampleTime=Ts_sample
  Selector : Selector  InputPortWidth=nObs  IndexOptions=Index vector (dialog)  Indices=1:2  OutputSizes=1
  Square{,2,4,7} (4 alike) : Math  Operator=square
  Terminator{,1..8} (9 alike) : Terminator
  Unit Delay1 : UnitDelay  SampleTime=-1  HasFrameUpgradeWarning=on
  reward : Outport
  each_reward : Outport  Port=2
  wires:
  action/1 -> Unit Delay1/1  "steering"
  Square2/1 -> Gain2/1
  Unit Delay1/1 -> Square2/1
  Demux2/2 -> Rate Transition7/1, Square7/1
  Square7/1 -> Gain5/1
  Square4/1 -> Gain4/1
  Add3/1 -> Exp/1
  obs/1 -> Selector/1
  Demux2/1 -> Rate Transition6/1, Square4/1
  Gain4/1 -> Add3/1
  Gain5/1 -> Add3/2
  Exp/1 -> Gain12/1
  Selector/1 -> Gain11/1
  Add2/1 -> Rate Transition8/1, Square/1  "th_err"
  Square/1 -> Gain/1
  Gain/1 -> Exp1/1
  Constant/1 -> Add2/2
  theta/1 -> Add2/1
  Exp1/1 -> Gain7/1
  Gain12/1 -> Rate Transition/1, Mux/1, Add/1
  Gain7/1 -> Rate Transition1/1, Mux/2, Add/2  "orient reward"
  Gain11/1 -> Demux2/1
  isParked/1 -> Rate Transition4/1, Gain1/1
  Gain1/1 -> Add/4  "parking reward"
  isInvalid/1 -> Rate Transition5/1, Gain3/1
  Gain3/1 -> Add/5  "collision penalty"
  Rate Transition/1 -> Terminator/1  "dist_reward"
  Rate Transition1/1 -> Terminator1/1  "orient_reward"
  Rate Transition2/1 -> Terminator2/1  "stable_reward"
  Gain2/1 -> Gain6/1
  Gain6/1 -> Mux/3, Add/3, Rate Transition2/1  "control penalty"
  Add/1 -> Rate Transition3/1, reward/1
  Rate Transition3/1 -> Terminator3/1  "reward"
  Rate Transition4/1 -> Terminator4/1  "is_parked"
  Rate Transition5/1 -> Terminator5/1  "is_collision"
  Rate Transition6/1 -> Terminator6/1  "x_error"
  Rate Transition7/1 -> Terminator7/1  "y_error"
  Rate Transition8/1 -> Terminator8/1  "theta_error"
  Mux/1 -> each_reward/1
  lidarMinDist/1 -> Compare To Constant/1
  Gain8/1 -> Add/6  "collision penalty"
  Compare To Constant/1 -> Gain8/1

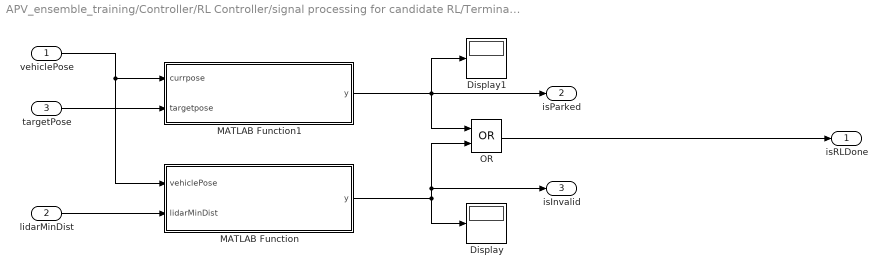
== system APV_ensemble_training/Controller/RL Controller/signal processing for candidate RL/Termination ==
  vehiclePose : Inport
  lidarMinDist : Inport  Port=2
  targetPose : Inport  Port=3
  Display : Display
  Display1 : Display
  MATLAB Function : MATLAB Function  TreatAsAtomicUnit=on
  MATLAB Function1 : MATLAB Function  TreatAsAtomicUnit=on
  OR : Logic  Operator=OR  AllPortsSameDT=off  OutDataTypeStr=boolean
  isRLDone : Outport
  isParked : Outport  Port=2
  isInvalid : Outport  Port=3
  wires:
  vehiclePose/1 -> MATLAB Function/1(vehiclePose), MATLAB Function1/1(currpose)
  lidarMinDist/1 -> MATLAB Function/2(lidarMinDist)
  OR/1 -> isRLDone/1
  targetPose/1 -> MATLAB Function1/2(targetpose)
  MATLAB Function1/1(y) -> Display1/1, isParked/1, OR/1
  MATLAB Function/1(y) -> OR/2, isInvalid/1, Display/1

== matlab function APV_ensemble_training/Controller/RL Controller/MATLAB Function ==
  data: u input; y output
function y = fcn(u)

if u ==0
    y= 1;
else
    y = u;
end

== matlab function APV_ensemble_training/Controller/RL Controller/Semantics Prediction/MATLAB Function ==
  data: allActions input; nextReward output; reward input; actionUB input; rewardUB_1 input; rewardUB_2 input; rewardToIndexTable input; tranTable input; stateTable input; actionTable input
function nextReward  = fcn(allActions, reward, actionUB, rewardUB_1,rewardUB_2, rewardToIndexTable, tranTable, stateTable,actionTable)

numController = 9;

nextReward = ones(numController, 1);
abReward_1 = find(rewardUB_1 >= reward(1), 1, 'first');  % concrete state -> abstract state
abReward_2 = find(rewardUB_2 >= reward(2), 1, 'first');

if isempty(abReward_1) || isempty(abReward_2)      % if this is an unseen reward
    nextReward = zeros(numController,1);
else
    rewardIndex1 = rewardToIndexTable(:,1)==abReward_1;
    rewardIndex2 = rewardToIndexTable(:,2)==abReward_2;
    
    if isempty(rewardIndex1) || isempty(rewardIndex2)      % if this is an unseen abstract state
        nextReward = zeros(numController,1);
    else
        abState = rewardToIndexTable(rewardToIndexTable(:,1)==abReward_1 & rewardToIndexTable(:,2)==abReward_2, 3);
        
        if isempty(abState)
            nextReward = zeros(numController,1);
        else
            for i = 1:numController
            
                action = allActions(i);
                abAction = find(actionUB >= action, 1, 'first');      % concrete action -> abstract action
            
                stateIndex = stateTable==abState;
                actionindex = actionTable==abAction;
            
                if isempty(stateIndex) || isempty(actionindex)  % if this is an unseen abstract state-action pair
                    abTranReward = 0;
                else
                    temp = stateIndex + actionindex;
                    if ismember(2,temp)
                        abTranReward = tranTable((stateIndex & actionindex),5);
                    else
                        abTranReward = 0;
                    end
                end
                nextReward(i,1) = abTranReward;
            end
        end
    end
end

== matlab function APV_ensemble_training/Controller/RL Controller/signal processing for candidate RL/Termination/MATLAB Function ==
  data: vehiclePose input; lidarMinDist input; y output; xBounds parameter; yBounds parameter; trainXBounds parameter; trainYBounds parameter; doTraining parameter; lidarTol parameter
function y = isOutOfBounds(vehiclePose, lidarMinDist, xBounds, yBounds, trainXBounds, trainYBounds, doTraining, lidarTol)

if doTraining
    xlims = trainXBounds;
    ylims = trainYBounds;
else
    xlims = xBounds;
    ylims = yBounds;
end

% get coordinates of four corners
xc = vehiclePose(1);
yc = vehiclePose(2);
t  = vehiclePose(3);

% threshold
tol = 0.1;

% Check if true positions are out of bounds
xOutOfBounds = xc <= xlims(1) + tol || xc >= xlims(2) - tol;
yOutOfBounds = yc <= ylims(1) + tol || yc >= ylims(2) - tol;

% check if lidar reading is less than threshold value
veryCloseToObstacle = lidarMinDist <= lidarTol;

goingInCircles = false;
if doTraining
    goingInCircles = t > 2*pi;
end

y = xOutOfBounds || yOutOfBounds || veryCloseToObstacle || goingInCircles;

== matlab function APV_ensemble_training/Controller/RL Controller/signal processing for candidate RL/Observations/MATLAB Function ==
  data: pose input; newpose output; targetposeidx input
function newpose = transformPose(pose,targetposeidx)
newpose = transformPose(pose,targetposeidx);

== matlab function APV_ensemble_training/Controller/RL Controller/signal processing for candidate RL/Lidar Processing/MATLAB Function ==
  data: carDistances output; W parameter; L parameter; res parameter
function carDistances = getDistances2CarBoundary(W,L,res)

angles = (0:(res-1))*2*pi/res;
carDistances = getCarSegmentLengths(L,W,angles);

== matlab function APV_ensemble_training/Controller/MPC Tracking Controller/Variant Subsystem/Nonlinear MPC/Reference Preview from RRT ==
  data: t input; ref output; Ts parameter; Tf parameter; pTracking parameter; Xref parameter
function ref = fcn(t,Ts,Tf,pTracking,Xref)
Tend = Tf;
T = t+(1:pTracking)*Ts;
T = min(T,Tend);
time = Ts*(1:length(Xref));
ref = interp1(time,Xref,T);

== matlab function APV_ensemble_training/Controller/RL Controller/signal processing for candidate RL/Termination/MATLAB Function1 ==
  data: currpose input; y output; targetpose input; xyerrTol parameter; terrTol parameter
function y = isParked(currpose,targetpose, xyerrTol, terrTol)

x = currpose(1);
y = currpose(2);
t = currpose(3);
xg = targetpose(1);
yg = targetpose(2);
tg = targetpose(3);
xyerr = sqrt((x-xg)^2+(y-yg)^2);
terr = wrapToPi(t)-tg;
y = 0;
if xyerr < xyerrTol && abs(terr) < terrTol
    y = 1;
end

== matlab function APV_ensemble_training/Controller/RL Controller/signal processing for candidate RL/Observations/MATLAB Function1 ==
  data: pose input; newpose output; targetposeidx input
function newpose = transformPose(pose,targetposeidx)
newpose = transformPose(pose,targetposeidx);

== matlab function APV_ensemble_training/Controller/MPC Tracking Controller/Variant Subsystem/Adaptive MPC/Plant Model Generator ==
  settings: updateMethod=DISCRETE  sampleTime=Ts
  data: x input size=[3,1]; u input size=[2,1]; A output; B output; C output; D output; U output size=[2,1]; Y output size=[3,1]; X output size=[3,1]; DX output size=[3,1]; Ts parameter
function [A,B,C,D,U,Y,X,DX] = fcn(x,u,Ts)

[A,B,C,D,U,Y,X,DX] = vehicleStateJacobianFcnDT(Ts,x,u);

== matlab function APV_ensemble_training/Controller/MPC Tracking Controller/Variant Subsystem/Adaptive MPC/Reference Preview from planner ==
  data: t input; ref output; Ts parameter; Tf parameter; pTracking parameter; Xref parameter
function ref = fcn(t,Ts,Tf,pTracking,Xref)
Tend = Tf;
T = t+(1:pTracking)*Ts;
T = min(T,Tend);
time = Ts*(1:length(Xref*1.2));
ref = interp1(time,Xref,T);
